simulink model "d_009_hvdc"  (Simulink 5.1)
settings: Solver=ode45  StartTime=0.0  StopTime=10.0  RelTol=1e-3
libraries: fm_lib x11
settings Model: Creator=fmilano  LastModifiedBy=fmilano  ExtModeAutoUpdateStatusClock=off  SignalLoggingName=logsout  RTWOptions="-aEnforceIntegerDowncast=1 -aFoldNonRolledExpr=1 -aInlineInvariantSignals=1 -aInlineParameters=0 -aLocalBlockOutputs=1 -aRollThreshold=5 -aZeroInternalMemoryAtStartup=1 -aZeroExternalMemoryAtStartup=1 -aInitFltsAndDblsToZero=1 -aForceBlockIOInitOptimize=0 -aGenerateReport=0 -aGenCodeOnly=0 -aRTWVerbose=1 -aIncludeHyperlinkInReport=0 -aLaunchReport=0 -aGenerateTraceInfo=0  -aForceParamTrailComments=0 -aGenerateComments=1 -aIgnoreCustomStorageClasses=1 -aIncHierarchyInIds=0 -aMaxRTWIdLen=31 -aShowEliminatedStatements=0 -aIncDataTypeInIds=0 -aInsertBlockDesc=0 -aIgnoreTestpoints=0 -aSimulinkBlockComments=1 -aInlinedPrmAccess=\"Literals\"  -aSuppressErrorStatus=0 -aModelReferenceCompliant=1 -aParenthesesLevel=\"Nominal\" -aModelStepFunctionPrototypeControlCompliant=0 -aPortableWordSizes=0 -aParMdlRefBuildCompliant=1 -aSupportNonInlinedSFcns=1 -aSupportContinuousTime=1 -aSupportComplex=1 -aSupportNonFinite=1 -aSupportAbsoluteTime=1 -aMultiwordLength=2048 -aTargetPreCompLibLocation=\"\" -aTargetLibSuffix=\"\" -aTargetFunctionLibrary=\"ANSI_C\" -aTargetFcnLib=\"ansi_tfl_tmw.mat\" -aMultiInstanceERTCode=0 -aLogVarNameModifier=\"rt_\" -aERTFirstTimeCompliant=0 -aIsPILTarget=0 -aCombineOutputUpdateFcns=0 -aGenerateASAP2=0 -aGenerateClassInterface=0 -aGenerateTestInterfaces=0 -aGenerateSampleERTMain=0 -aGenerateFullHeader=1 -aUtilityFuncGeneration=\"Auto\" -aIncludeFileDelimiter=\"Auto\" -aIncludeMdlTerminateFcn=1 -aPurelyIntegerCode=0 -aAutosarCompliant=0 -aERTCustomFileBanners=0 -aRTWCAPIStates=0 -aRTWCAPIParams=0 -aRTWCAPISignals=0 -aMatFileLogging=1 -aCompOptLevelCompliant=0 -aCPPClassGenCompliant=0 -aExtModeIntrfLevel=\"Level1\" -aExtModeMexFile=\"ext_comm\" -aExtModeTransport=0 -aExtModeStaticAllocSize=1000000 -aExtModeTesting=0 -aExtModeStaticAlloc=0 -aExtMode=0 -aERTMultiwordLength=256 -aERTMultiwordTypeDef=\"System defined\"  -aGenerateTraceInfo=0 -aIgnoreTestpoints=0 -aGenerateTraceInfo=0 -aGenerateTraceInfo=0 -aGenerateTraceInfo=0 -aGenerateTraceInfo=0 -aPrefixModelToSubsysFcnNames=1"

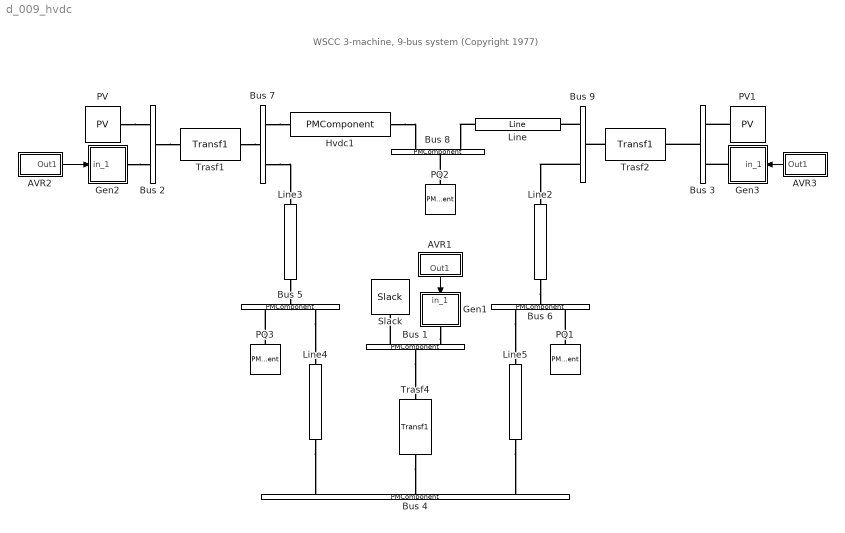
== system d_009_hvdc ==
  note: WSCC 3-machine, 9-bus system (Copyright 1977)
  AVR1 : Subsystem  Tag=PSATblock  Description=Controls  Orientation=down  mask(Exc){p2q=2, p3q=5.00, p4q=-5.00, p5q=20, p6q=0.2, p7q=0.063, p8q=0.35, p9q=1, p10q=0.314, p11q=0.001, p12_13q=[0.0039  1.555], in=0}
      mask prompts: p2q "Automatic Voltage Regulator Type"; p3q "Maximum Regulator Voltage [p.u.]"; p4q "Minimum Regulator Voltage [p.u.]"; p5q "Amplifier Gain Ka [p.u./p.u.]"; p6q "Amplifier Time Constant Ta [s]"; p7q "Stabilizer Gain Kf [p.u./p.u.]"; p8q "Stabilizer Time Tf [s]"; p9q "Integral deviation Ke [p.u./p.u.]"; p10q "Time Constant of the Field Circuit Td [s]"; p11q "Time Delay of the Measurement System Tr [s]"; p12_13q "Coefficient of the Ceiling Function (A B)"; in "Number of input signals"
      mask help: This block defines an Automatic Voltage Regulator.
      mask init:
      | fm_inout
      | [x,y] = fm_draw('R');
      mask Help:
      | This block defines an Automatic Voltage Regulator.
      | There are three kind of regulators:
      | 
      | Type 1:
      | 
      |      IEEE Model 1
      | 
      | Type 2:
      | 
      |      IEEE Model 2
      | 
      | Type 3:
      | 
      |      IEEE Model 3
      mask StyleString: popup(1|2|3),edit,edit,edit,edit,edit,edit,edit,edit,edit,edit,popup(0|1|2|3)
      mask CallbackString: fm_block|||||||||||
      mask Display:
      | plot([-1.8 4.1 4.1 -1.8 -1.8],[-1.5 -1.5 1.5 1.5 -1.5])
      | color('red')
      | plot([-1.3 -0.5],[-1 1],[-0.5 0.3],[1 -1],[-0.9 -0.1],[0.0 0.0])
      | plot(2.8+1.3*x,2*y,1.5+[-1.3 -0.5],[1 -1],1.5+[-0.5 0.3],[-1 1])
  AVR2 : Subsystem  Tag=PSATblock  Description=Controls  mask(Exc){p2q=2, p3q=5.00, p4q=-5.00, p5q=20, p6q=0.2, p7q=0.063, p8q=0.35, p9q=1, p10q=0.314, p11q=0.001, p12_13q=[0.0039  1.555], in=0}
      mask prompts: p2q "Automatic Voltage Regulator Type"; p3q "Maximum Regulator Voltage [p.u.]"; p4q "Minimum Regulator Voltage [p.u.]"; p5q "Amplifier Gain Ka [p.u./p.u.]"; p6q "Amplifier Time Constant Ta [s]"; p7q "Stabilizer Gain Kf [p.u./p.u.]"; p8q "Stabilizer Time Tf [s]"; p9q "Integral deviation Ke [p.u./p.u.]"; p10q "Time Constant of the Field Circuit Td [s]"; p11q "Time Delay of the Measurement System Tr [s]"; p12_13q "Coefficient of the Ceiling Function (A B)"; in "Number of input signals"
      mask help: This block defines an Automatic Voltage Regulator.
      mask init:
      | fm_inout
      | [x,y] = fm_draw('R');
      mask Help:
      | This block defines an Automatic Voltage Regulator.
      | There are three kind of regulators:
      | 
      | Type 1:
      | 
      |      IEEE Model 1
      | 
      | Type 2:
      | 
      |      IEEE Model 2
      | 
      | Type 3:
      | 
      |      IEEE Model 3
      mask StyleString: popup(1|2|3),edit,edit,edit,edit,edit,edit,edit,edit,edit,edit,popup(0|1|2|3)
      mask CallbackString: fm_block|||||||||||
      mask Display:
      | plot([-1.8 4.1 4.1 -1.8 -1.8],[-1.5 -1.5 1.5 1.5 -1.5])
      | color('red')
      | plot([-1.3 -0.5],[-1 1],[-0.5 0.3],[1 -1],[-0.9 -0.1],[0.0 0.0])
      | plot(2.8+1.3*x,2*y,1.5+[-1.3 -0.5],[1 -1],1.5+[-0.5 0.3],[-1 1])
  AVR3 : Subsystem  Tag=PSATblock  Description=Controls  Orientation=left  mask(Exc){p2q=2, p3q=5.00, p4q=-5.00, p5q=20, p6q=0.2, p7q=0.063, p8q=0.35, p9q=1, p10q=0.314, p11q=0.001, p12_13q=[0.0039  1.555], in=0}
      mask prompts: p2q "Automatic Voltage Regulator Type"; p3q "Maximum Regulator Voltage [p.u.]"; p4q "Minimum Regulator Voltage [p.u.]"; p5q "Amplifier Gain Ka [p.u./p.u.]"; p6q "Amplifier Time Constant Ta [s]"; p7q "Stabilizer Gain Kf [p.u./p.u.]"; p8q "Stabilizer Time Tf [s]"; p9q "Integral deviation Ke [p.u./p.u.]"; p10q "Time Constant of the Field Circuit Td [s]"; p11q "Time Delay of the Measurement System Tr [s]"; p12_13q "Coefficient of the Ceiling Function (A B)"; in "Number of input signals"
      mask help: This block defines an Automatic Voltage Regulator.
      mask init:
      | fm_inout
      | [x,y] = fm_draw('R');
      mask Help:
      | This block defines an Automatic Voltage Regulator.
      | There are three kind of regulators:
      | 
      | Type 1:
      | 
      |      IEEE Model 1
      | 
      | Type 2:
      | 
      |      IEEE Model 2
      | 
      | Type 3:
      | 
      |      IEEE Model 3
      mask StyleString: popup(1|2|3),edit,edit,edit,edit,edit,edit,edit,edit,edit,edit,popup(0|1|2|3)
      mask CallbackString: fm_block|||||||||||
      mask Display:
      | plot([-1.8 4.1 4.1 -1.8 -1.8],[-1.5 -1.5 1.5 1.5 -1.5])
      | color('red')
      | plot([-1.3 -0.5],[-1 1],[-0.5 0.3],[1 -1],[-0.9 -0.1],[0.0 0.0])
      | plot(2.8+1.3*x,2*y,1.5+[-1.3 -0.5],[1 -1],1.5+[-0.5 0.3],[-1 1])
  Bus 1 : PMComponent  Tag=PSATblock  Description=Connection  Orientation=down  PhysicalDomain=psatdomain  LeftPortType=p1  RightPortType=p1  LConnTagsString=__newl0|__newl1  RConnTagsString=__newr0  mask(Bus){in=2, out=1, p2q=16.5, p3_4q=[1.00   0.00], p5q=4, p6q=1}
      mask prompts: in "Number of inputs:"; out "Number of outputs:"; p2q "Voltage Rating [kV]"; p3_4q "Voltage initial guess [p.u.  rad]"; p5q "Area number"; p6q "Region number"
      mask help: Bus block.
      mask init:
      | fm_inout
      mask CallbackString: ||||fm_block|
      mask Display: plot([0 1 1 0 0],[0 0 1 1 0])
  Bus 2 : PMComponent  Tag=PSATblock  Description=Connection  PhysicalDomain=psatdomain  LeftPortType=p1  RightPortType=p1  LConnTagsString=__newl0|__newl1  RConnTagsString=__newr0  mask(Bus){in=2, out=1, p2q=18, p3_4q=[1.00   0.00], p5q=5, p6q=1}
      mask prompts: in "Number of inputs:"; out "Number of outputs:"; p2q "Voltage Rating [kV]"; p3_4q "Voltage initial guess [p.u.  rad]"; p5q "Area number"; p6q "Region number"
      mask help: Bus block.
      mask init:
      | fm_inout
      mask CallbackString: ||||fm_block|
      mask Display: plot([0 1 1 0 0],[0 0 1 1 0])
  Bus 3 : PMComponent  Tag=PSATblock  Description=Connection  Orientation=left  PhysicalDomain=psatdomain  LeftPortType=p1  RightPortType=p1  LConnTagsString=__newl0|__newl1  RConnTagsString=__newr0  mask(Bus){in=2, out=1, p2q=13.8, p3_4q=[1.00   0.00], p5q=3, p6q=1}
      mask prompts: in "Number of inputs:"; out "Number of outputs:"; p2q "Voltage Rating [kV]"; p3_4q "Voltage initial guess [p.u.  rad]"; p5q "Area number"; p6q "Region number"
      mask help: Bus block.
      mask init:
      | fm_inout
      mask CallbackString: ||||fm_block|
      mask Display: plot([0 1 1 0 0],[0 0 1 1 0])
  Bus 4 : PMComponent  Tag=PSATblock  Description=Connection  Orientation=down  PhysicalDomain=psatdomain  LeftPortType=p1  RightPortType=p1  LConnTagsString=__newl0|__newl1|__newl2  mask(Bus){in=3, out=0, p2q=230, p3_4q=[1.00   0.00], p5q=2, p6q=1}
      mask prompts: in "Number of inputs:"; out "Number of outputs:"; p2q "Voltage Rating [kV]"; p3_4q "Voltage initial guess [p.u.  rad]"; p5q "Area number"; p6q "Region number"
      mask help: Bus block.
      mask init:
      | fm_inout
      mask CallbackString: ||||fm_block|
      mask Display: plot([0 1 1 0 0],[0 0 1 1 0])
  Bus 5 : PMComponent  Tag=PSATblock  Description=Connection  Orientation=down  PhysicalDomain=psatdomain  LeftPortType=p1  RightPortType=p1  LConnTagsString=__newl0  RConnTagsString=__newr0|__newr1  mask(Bus){in=1, out=2, p2q=230, p3_4q=[1.00   0.00], p5q=2, p6q=1}
      mask prompts: in "Number of inputs:"; out "Number of outputs:"; p2q "Voltage Rating [kV]"; p3_4q "Voltage initial guess [p.u.  rad]"; p5q "Area number"; p6q "Region number"
      mask help: Bus block.
      mask init:
      | fm_inout
      mask CallbackString: ||||fm_block|
      mask Display: plot([0 1 1 0 0],[0 0 1 1 0])
  Bus 6 : PMComponent  Tag=PSATblock  Description=Connection  Orientation=down  PhysicalDomain=psatdomain  LeftPortType=p1  RightPortType=p1  LConnTagsString=__newl0  RConnTagsString=__newr0|__newr1  mask(Bus){in=1, out=2, p2q=230, p3_4q=[1.00   0.00], p5q=2, p6q=1}
      mask prompts: in "Number of inputs:"; out "Number of outputs:"; p2q "Voltage Rating [kV]"; p3_4q "Voltage initial guess [p.u.  rad]"; p5q "Area number"; p6q "Region number"
      mask help: Bus block.
      mask init:
      | fm_inout
      mask CallbackString: ||||fm_block|
      mask Display: plot([0 1 1 0 0],[0 0 1 1 0])
  Bus 7 : PMComponent  Tag=PSATblock  Description=Connection  PhysicalDomain=psatdomain  LeftPortType=p1  RightPortType=p1  LConnTagsString=__newl0  RConnTagsString=__newr0|__newr1  mask(Bus){in=1, out=2, p2q=230, p3_4q=[1.00   0.00], p5q=2, p6q=1}
      mask prompts: in "Number of inputs:"; out "Number of outputs:"; p2q "Voltage Rating [kV]"; p3_4q "Voltage initial guess [p.u.  rad]"; p5q "Area number"; p6q "Region number"
      mask help: Bus block.
      mask init:
      | fm_inout
      mask CallbackString: ||||fm_block|
      mask Display: plot([0 1 1 0 0],[0 0 1 1 0])
  Bus 8 : PMComponent  Tag=PSATblock  Description=Connection  Orientation=down  PhysicalDomain=psatdomain  LeftPortType=p1  RightPortType=p1  LConnTagsString=__newl0|__newl1  RConnTagsString=__newr0  mask(Bus){in=2, out=1, p2q=230, p3_4q=[1.00   0.00], p5q=2, p6q=1}
      mask prompts: in "Number of inputs:"; out "Number of outputs:"; p2q "Voltage Rating [kV]"; p3_4q "Voltage initial guess [p.u.  rad]"; p5q "Area number"; p6q "Region number"
      mask help: Bus block.
      mask init:
      | fm_inout
      mask CallbackString: ||||fm_block|
      mask Display: plot([0 1 1 0 0],[0 0 1 1 0])
  Bus 9 : PMComponent  Tag=PSATblock  Description=Connection  Orientation=left  PhysicalDomain=psatdomain  LeftPortType=p1  RightPortType=p1  LConnTagsString=__newl0  RConnTagsString=__newr0|__newr1  mask(Bus){in=1, out=2, p2q=230, p3_4q=[1.00   0.00], p5q=2, p6q=1}
      mask prompts: in "Number of inputs:"; out "Number of outputs:"; p2q "Voltage Rating [kV]"; p3_4q "Voltage initial guess [p.u.  rad]"; p5q "Area number"; p6q "Region number"
      mask help: Bus block.
      mask init:
      | fm_inout
      mask CallbackString: ||||fm_block|
      mask Display: plot([0 1 1 0 0],[0 0 1 1 0])
  Gen1 : Subsystem  Tag=PSATblock  Description=Machines  Orientation=down  mask(Syn){p2_3_4q=[100  16.5   60], p5q=4, p7_6q=[0.00  0.00], p8_9_10q=[0.1460  0.0608  0.0000], p11_12q=[8.96  0.00], p13_14_15q=[0.0969  0.0969  0.0000], p16_17q=[0.310  0.0000], p18_19q=[2*23.64  0.00], p20_21q=[0.00  0.00], p22_23q=[1.00  1.00], p24q=0.002, p25_26q=[0 0], in=1}
      mask prompts: p2_3_4q "Power, voltage and frequency ratings [MVA, kV, Hz]"; p5q "Machine Dynamic Order"; p7_6q "resistance ra and leakage reactance xl [p.u. p.u.]"; p8_9_10q "d-axis reactances Xd, X'd X"d [p.u.,p.u.,p.u.]"; p11_12q "d-axis open circuit time constants T'd0 and T"d0 [s, s]"; p13_14_15q "q-axis reactances Xq, X'q, X"q [p.u.  p.u.  p.u.]"; p16_17q "q-axis open circuit time constants T'q0 and T"q0 [s s]"; p18_19q "Inertia (M = 2H) and Damping [s, p.u.]"; p20_21q "Speed and active power additional signals Kw & Kp [p.u., p.u.]"; p22_23q "Percentage of active and reactive powers at bus [p.u. p.u.]"; p24q "d-axis additional circuit leakage time constant Taa [s]"; p25_26q "Saturation coefficients S(1.0) and S(1.2)"; in "Number of input signals"
      mask help: This block defines a fourth order synchronous machine.
      mask init:
      | fm_inout
      | [x,y] = fm_draw('circle');
      | [xg,yg] = fm_draw('G');
      | [xs,ys] = fm_draw('sinus');
      mask StyleString: edit,popup(8|6|5.3|5.2|5.1|4|3|2),edit,edit,edit,edit,edit,edit,edit,edit,edit,edit,popup(0|1|2)
      mask CallbackString: |fm_block|||||||||||
      mask Display:
      | plot(x+1.4,y,0.12*xs+1,0.15*ys-0.6)
      | color('blue')
      | plot(1.4+0.45*xg,0.3+0.45*yg)
  Gen2 : Subsystem  Tag=PSATblock  Description=Machines  mask(Syn){p2_3_4q=[100  18   60], p5q=4, p7_6q=[0.00  0.00], p8_9_10q=[0.8958  0.1198  0.0000], p11_12q=[6.00  0.00], p13_14_15q=[0.8645  0.1969  0.0000], p16_17q=[0.5350  0.0000], p18_19q=[12.80  0.00], p20_21q=[0.00  0.00], p22_23q=[1.00  1.00], p24q=0.002, p25_26q=[0 0], in=1}
      mask prompts: p2_3_4q "Power, voltage and frequency ratings [MVA, kV, Hz]"; p5q "Machine Dynamic Order"; p7_6q "resistance ra and leakage reactance xl [p.u. p.u.]"; p8_9_10q "d-axis reactances Xd, X'd X"d [p.u.,p.u.,p.u.]"; p11_12q "d-axis open circuit time constants T'd0 and T"d0 [s, s]"; p13_14_15q "q-axis reactances Xq, X'q, X"q [p.u.  p.u.  p.u.]"; p16_17q "q-axis open circuit time constants T'q0 and T"q0 [s s]"; p18_19q "Inertia (M = 2H) and Damping [s, p.u.]"; p20_21q "Speed and active power additional signals Kw & Kp [p.u., p.u.]"; p22_23q "Percentage of active and reactive powers at bus [p.u. p.u.]"; p24q "d-axis additional circuit leakage time constant Taa [s]"; p25_26q "Saturation coefficients S(1.0) and S(1.2)"; in "Number of input signals"
      mask help: This block defines a fourth order synchronous machine.
      mask init:
      | fm_inout
      | [x,y] = fm_draw('circle');
      | [xg,yg] = fm_draw('G');
      | [xs,ys] = fm_draw('sinus');
      mask StyleString: edit,popup(8|6|5.3|5.2|5.1|4|3|2),edit,edit,edit,edit,edit,edit,edit,edit,edit,edit,popup(0|1|2)
      mask CallbackString: |fm_block|||||||||||
      mask Display:
      | plot(x+1.4,y,0.12*xs+1,0.15*ys-0.6)
      | color('blue')
      | plot(1.4+0.45*xg,0.3+0.45*yg)
  Gen3 : Subsystem  Tag=PSATblock  Description=Machines  Orientation=left  mask(Syn){p2_3_4q=[100  13.8   60], p5q=4, p7_6q=[0.00  0.00], p8_9_10q=[1.3125  0.1813  0.0000], p11_12q=[5.89  0.00], p13_14_15q=[1.2578  0.2500  0.0000], p16_17q=[0.600  0.0000], p18_19q=[6.02  0.00], p20_21q=[0.00  0.00], p22_23q=[1.00  1.00], p24q=0.002, p25_26q=[0 0], in=1}
      mask prompts: p2_3_4q "Power, voltage and frequency ratings [MVA, kV, Hz]"; p5q "Machine Dynamic Order"; p7_6q "resistance ra and leakage reactance xl [p.u. p.u.]"; p8_9_10q "d-axis reactances Xd, X'd X"d [p.u.,p.u.,p.u.]"; p11_12q "d-axis open circuit time constants T'd0 and T"d0 [s, s]"; p13_14_15q "q-axis reactances Xq, X'q, X"q [p.u.  p.u.  p.u.]"; p16_17q "q-axis open circuit time constants T'q0 and T"q0 [s s]"; p18_19q "Inertia (M = 2H) and Damping [s, p.u.]"; p20_21q "Speed and active power additional signals Kw & Kp [p.u., p.u.]"; p22_23q "Percentage of active and reactive powers at bus [p.u. p.u.]"; p24q "d-axis additional circuit leakage time constant Taa [s]"; p25_26q "Saturation coefficients S(1.0) and S(1.2)"; in "Number of input signals"
      mask help: This block defines a fourth order synchronous machine.
      mask init:
      | fm_inout
      | [x,y] = fm_draw('circle');
      | [xg,yg] = fm_draw('G');
      | [xs,ys] = fm_draw('sinus');
      mask StyleString: edit,popup(8|6|5.3|5.2|5.1|4|3|2),edit,edit,edit,edit,edit,edit,edit,edit,edit,edit,popup(0|1|2)
      mask CallbackString: |fm_block|||||||||||
      mask Display:
      | plot(x+1.4,y,0.12*xs+1,0.15*ys-0.6)
      | color('blue')
      | plot(1.4+0.45*xg,0.3+0.45*yg)
  Hvdc1 : PMComponent  Tag=PSATblock  Description=FACTS  PhysicalDomain=psatdomain  LeftPortType=p1  RightPortType=p1  LConnTagsString=__newl0  RConnTagsString=__newr0  mask(Hvdc){p3_6q=[100  60], p4_5q=[230 230], p7_8q=[300 0.3], p9_10q=[0.1345   0.1257], p11_12q=[0.975  0.975], p13_14q=[20  25], p15_16q=[0.0625  0.200], p17_18q=[120  5], p19_20q=[40  18], p21_22_23_24q=[1.2   0.1  1.1  0.0], p25q=Current_control, p26_27_28q=[1  0.5  1.0], p29q=on}
      mask prompts: p3_6q "Power and Frequency Ratings [MVA,  Hz]"; p4_5q "Voltage Rating at Terminal Buses [kV, kV]"; p7_8q "DC Ratings (Vn_dc, In_dc) [kV, kA]"; p9_10q "Transformer Reactances (Xcr  Xci) [p.u.  p.u.]"; p11_12q "Tap Ratios (Ar Ai) [p.u./p.u.  p.u./p.u.]"; p13_14q "PI Regulator Constants (Ki, Kp)"; p15_16q "DC Line Parameters (Rdc Ldc) [p.u.  p.u.]"; p17_18q "Rectifier Angle Limits (a_max, a_min) [deg  deg]"; p19_20q "Inverter Angle Limits (g_max, g_min) [deg  deg]"; p21_22_23_24q "Reference dc voltage limits (Vr_max, Vr_min, Vi_max, Vi_min) [p.u.]"; p25q "Control type"; p26_27_28q "Current, active power and dc voltage orders [p.u.  p.u.  p.u.]"; p29q "Connected"
      mask help: This block defines a HVDC connection.
      mask init:
      | [x,y] = fm_draw('circle');
      mask StyleString: edit,edit,edit,edit,edit,edit,edit,edit,edit,edit,popup(Current_control|Power_control|Voltage_control),edit,checkbox
      mask CallbackString: ||||||||||||fm_block
      mask Display:
      | plot(0.7+[0 4 4 0 0],[-2 -2 2 2 -2])
      | plot(9.7+[0 4 4 0 0],[-2 -2 2 2 -2])
      | plot([4.7 9.7],[-1.25 -1.25],[4.7 9.7],[1.25 1.25])
      | 
      | plot(x-2,y,x-0.6,y,x+15,y,x+16.4,y)
      | color('green')
      | plot(-2+[-1 -1.3],[0 0],-2+[2.4 2.7],[0 0])
      | plot(-2+[-0.8 0.7],[-1.2 1.2],-2+[0.5 0.7],[1.1 1.2],-2+[0.7 0.7],[1.0 1.2])
      | plot(15+[-1 -1.3],[0 0],15+[2.4 2.7],[0 0])
      | plot(16.4+[-0.8 0.7],[-1.2 1.2],16.4+[0.5 0.7],[1.1 1.2],16.4+[0.7 0.7],[1.0 1.2])
      | 
      | color('magenta')
      | text(1.1,1.2,'R')
      | text(10.1,1.2,'I')
      | plot(0.7+[1 3 2 1],[-0.9 -0.9 0.9 -0.9])
      | plot(9.7+[1 3 2 1],[-0.9 -0.9 0.9 -0.9])
      | plot(0.7+[2 2],[0.9 1.25],0.7+[2 2],[-0.9 -1.25],0.7+[1.2 2.8],[0.9 0.9])
      | plot(9.7+[2 2],[0.9 1.25],9.7+[2 2],[-0.9 -1.25],9.7+[1.2 2.8],[0.9 0.9])
      | plot(0.7+[2 2.5],[0.9 1.25],9.7+[2 2.5],[0.9 1.25])
  Line : fm_lib/Power Flow/Line  Tag=PSATblock  Description=Power Flow  Orientation=left  PhysicalDomain=psatdomain  SubClassName=unknown  LeftPortType=p1  RightPortType=p1  LConnTagsString=__newl0  RConnTagsString=__newr0  p3_4_5q="[100  230  60]"  p6q=0  p8q=0.0119  p9q=0.1008  p10q=0.1045*2  p13_14_15q="[0.0  0.0  0.0]"  p16q=on
  Line2 : fm_lib/Power Flow/Line  Tag=PSATblock  Description=Power Flow  Orientation=down  PhysicalDomain=psatdomain  SubClassName=unknown  LeftPortType=p1  RightPortType=p1  LConnTagsString=__newl0  RConnTagsString=__newr0  p3_4_5q="[100  230  60]"  p6q=0  p8q=0.039  p9q=0.170  p10q=0.179*2  p13_14_15q="[0.0  0.0  0.0]"  p16q=on
  Line3 : fm_lib/Power Flow/Line  Tag=PSATblock  Description=Power Flow  Orientation=down  PhysicalDomain=psatdomain  SubClassName=unknown  LeftPortType=p1  RightPortType=p1  LConnTagsString=__newl0  RConnTagsString=__newr0  p3_4_5q="[100  230  60]"  p6q=0  p8q=0.032  p9q=0.161  p10q=0.153*2  p13_14_15q="[0.0  0.0  0.0]"  p16q=on
  Line4 : fm_lib/Power Flow/Line  Tag=PSATblock  Description=Power Flow  Orientation=down  PhysicalDomain=psatdomain  SubClassName=unknown  LeftPortType=p1  RightPortType=p1  LConnTagsString=__newl0  RConnTagsString=__newr0  p3_4_5q="[100  230  60]"  p6q=0  p8q=0.01  p9q=0.085  p10q=0.088*2  p13_14_15q="[0.0  0.0  0.0]"  p16q=on
  Line5 : fm_lib/Power Flow/Line  Tag=PSATblock  Description=Power Flow  Orientation=down  PhysicalDomain=psatdomain  SubClassName=unknown  LeftPortType=p1  RightPortType=p1  LConnTagsString=__newl0  RConnTagsString=__newr0  p3_4_5q="[100  230  60]"  p6q=0  p8q=0.017  p9q=0.092  p10q=0.079*2  p13_14_15q="[0.0  0.0  0.0]"  p16q=on
  PQ1 : PMComponent  Tag=PSATblock  Description=Power Flow  Orientation=down  PhysicalDomain=psatdomain  LeftPortType=p1  RightPortType=p1  LConnTagsString=__newl0  mask(PQ){p2_3q=[100  230], p4_5q=[0.90  0.30], p6_7q=[1.2  0.8], p8q=off, p9q=on}
      mask prompts: p2_3q "Power and Voltage Ratings [MVA, kV]"; p4_5q "Active and Reactive Powers [p.u.  p.u.]"; p6_7q "Maximum and Minimum Allowable Voltage [p.u.   p.u.]"; p8q "Allow conversion to impendance for min & max voltage"; p9q "Connected"
      mask help:
      | This block defines a constant power load:
      |
      | P = Pcost.
      | Q = Qcost.
      mask CallbackString: |||fm_block|fm_block
      mask Display: plot([1 -0.5 -0.5 1],[0 0.866 -0.866 0])
  PQ2 : PMComponent  Tag=PSATblock  Description=Power Flow  Orientation=down  PhysicalDomain=psatdomain  LeftPortType=p1  RightPortType=p1  LConnTagsString=__newl0  mask(PQ){p2_3q=[100  230], p4_5q=[1.00  0.35], p6_7q=[1.2  0.8], p8q=off, p9q=on}
      mask prompts: p2_3q "Power and Voltage Ratings [MVA, kV]"; p4_5q "Active and Reactive Powers [p.u.  p.u.]"; p6_7q "Maximum and Minimum Allowable Voltage [p.u.   p.u.]"; p8q "Allow conversion to impendance for min & max voltage"; p9q "Connected"
      mask help:
      | This block defines a constant power load:
      |
      | P = Pcost.
      | Q = Qcost.
      mask CallbackString: |||fm_block|fm_block
      mask Display: plot([1 -0.5 -0.5 1],[0 0.866 -0.866 0])
  PQ3 : PMComponent  Tag=PSATblock  Description=Power Flow  Orientation=down  PhysicalDomain=psatdomain  LeftPortType=p1  RightPortType=p1  LConnTagsString=__newl0  mask(PQ){p2_3q=[100  230], p4_5q=[1.25  0.50], p6_7q=[1.2  0.8], p8q=off, p9q=on}
      mask prompts: p2_3q "Power and Voltage Ratings [MVA, kV]"; p4_5q "Active and Reactive Powers [p.u.  p.u.]"; p6_7q "Maximum and Minimum Allowable Voltage [p.u.   p.u.]"; p8q "Allow conversion to impendance for min & max voltage"; p9q "Connected"
      mask help:
      | This block defines a constant power load:
      |
      | P = Pcost.
      | Q = Qcost.
      mask CallbackString: |||fm_block|fm_block
      mask Display: plot([1 -0.5 -0.5 1],[0 0.866 -0.866 0])
  PV : fm_lib/Power Flow/PV  Tag=PSATblock  Description=Power Flow  PhysicalDomain=psatdomain  SubClassName=unknown  LeftPortType=p1  RightPortType=p1  RConnTagsString=__newr0  p2_3q="[100  18]"  p4q=1.63  p5q=1.025  p6_7q=[99 -99]  p8_9q="[1.1  0.9]"  p10q=1  p11q=on
  PV1 : fm_lib/Power Flow/PV  Tag=PSATblock  Description=Power Flow  Orientation=left  PhysicalDomain=psatdomain  SubClassName=unknown  LeftPortType=p1  RightPortType=p1  RConnTagsString=__newr0  p2_3q="[100  13.8]"  p4q=0.85  p5q=1.025  p6_7q="[99  -99]"  p8_9q="[1.1  0.9]"  p10q=1  p11q=on
  Slack : fm_lib/Power Flow/Slack  Tag=PSATblock  Description=Power Flow  Orientation=down  PhysicalDomain=psatdomain  SubClassName=unknown  LeftPortType=p1  RightPortType=p1  RConnTagsString=__newr0  p2_3q="[100  16.5]"  p4q=1.04  p5q=0.00  p6_7q=[99 -99]  p8_9q="[1.1  0.9]"  p10q=0.80  p11q=1  p12q=on  p13q=on
  Trasf1 : fm_lib/Power Flow/Transf1  Tag=PSATblock  Description=Power Flow  PhysicalDomain=psatdomain  SubClassName=unknown  LeftPortType=p1  RightPortType=p1  LConnTagsString=__newl0  RConnTagsString=__newr0  p3_4_5q="[100  18  60]"  p7q=18/230  p8q=0.0  p9q=0.0625  p13_14_15q="[0.0  0.0  0.0]"  p16q=on
  Trasf2 : fm_lib/Power Flow/Transf1  Tag=PSATblock  Description=Power Flow  Orientation=left  PhysicalDomain=psatdomain  SubClassName=unknown  LeftPortType=p1  RightPortType=p1  LConnTagsString=__newl0  RConnTagsString=__newr0  p3_4_5q="[100  13.8  60]"  p7q=13.8/230  p8q=0.0  p9q=0.0586  p13_14_15q="[0.0  0.0  0.0]"  p16q=on
  Trasf4 : fm_lib/Power Flow/Transf1  Tag=PSATblock  Description=Power Flow  Orientation=down  PhysicalDomain=psatdomain  SubClassName=unknown  LeftPortType=p1  RightPortType=p1  LConnTagsString=__newl0  RConnTagsString=__newr0  p3_4_5q="[100  16.5  60]"  p7q=16.5/230  p8q=0.0  p9q=0.0576  p13_14_15q="[0.0  0.0  0.0]"  p16q=on
  wires:
  AVR2/1(Out1) -> Gen2/1(in_1)
  AVR3/1(Out1) -> Gen3/1(in_1)
  AVR1/1(Out1) -> Gen1/1(in_1)
  connections:
  Bus 7/RConn2 -- Line3/LConn1
  Gen1/RConn1 -- Bus 1/LConn2
  Gen3/RConn1 -- Bus 3/LConn2
  Gen2/RConn1 -- Bus 2/LConn2
  Bus 1/RConn1 -- Trasf4/LConn1
  Trasf4/RConn1 -- Bus 4/LConn2
  Line5/RConn1 -- Bus 4/LConn3
  Line4/RConn1 -- Bus 4/LConn1
  Bus 5/RConn2 -- Line4/LConn1
  Bus 6/RConn1 -- Line5/LConn1
  Line3/RConn1 -- Bus 5/LConn1
  Line2/RConn1 -- Bus 6/LConn1
  Bus 9/RConn2 -- Line2/LConn1
  Line/RConn1 -- Bus 8/LConn2
  Bus 7/RConn1 -- Hvdc1/LConn1
  Bus 9/RConn1 -- Line/LConn1
  Trasf2/RConn1 -- Bus 9/LConn1
  Trasf1/RConn1 -- Bus 7/LConn1
  Bus 3/RConn1 -- Trasf2/LConn1
  Bus 2/RConn1 -- Trasf1/LConn1
  PV1/RConn1 -- Bus 3/LConn1
  PV/RConn1 -- Bus 2/LConn1
  PQ1/LConn1 -- Bus 6/RConn2
  PQ2/LConn1 -- Bus 8/RConn1
  PQ3/LConn1 -- Bus 5/RConn1
  Bus 1/LConn1 -- Slack/RConn1
  Hvdc1/RConn1 -- Bus 8/LConn1

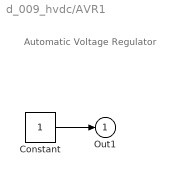
== system d_009_hvdc/AVR1 ==
  note: Automatic Voltage Regulator
  Constant : Constant  OutDataType=sfix(16)  OutScaling=2^0
  Out1 : Outport
  wires:
  Constant/1 -> Out1/1

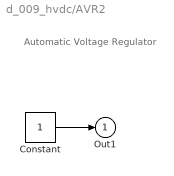
== system d_009_hvdc/AVR2 ==
  note: Automatic Voltage Regulator
  Constant : Constant  OutDataType=sfix(16)  OutScaling=2^0
  Out1 : Outport
  wires:
  Constant/1 -> Out1/1

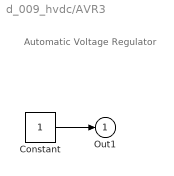
== system d_009_hvdc/AVR3 ==
  note: Automatic Voltage Regulator
  Constant : Constant  OutDataType=sfix(16)  OutScaling=2^0
  Out1 : Outport
  wires:
  Constant/1 -> Out1/1

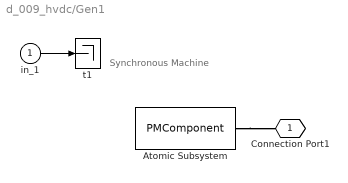
== system d_009_hvdc/Gen1 ==
  note: Synchronous Machine
  in_1 : Inport  OutDataType=sfix(16)  OutScaling=2^0
  Atomic Subsystem : PMComponent  PhysicalDomain=psatdomain  LeftPortType=p1  RightPortType=p1  RConnTagsString=__newr0
  t1 : Terminator
  Connection Port1 : PMIOPort  Tag=PMCPort  Orientation=left  Port=1  Side=Right
  wires:
  in_1/1 -> t1/1
  connections:
  Atomic Subsystem/RConn1 -- Connection Port1/RConn1

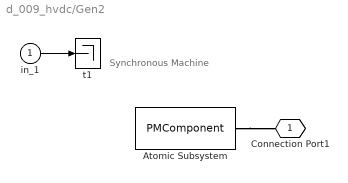
== system d_009_hvdc/Gen2 ==
  note: Synchronous Machine
  in_1 : Inport  OutDataType=sfix(16)  OutScaling=2^0
  Atomic Subsystem : PMComponent  PhysicalDomain=psatdomain  LeftPortType=p1  RightPortType=p1  RConnTagsString=__newr0
  t1 : Terminator
  Connection Port1 : PMIOPort  Tag=PMCPort  Orientation=left  Port=1  Side=Right
  wires:
  in_1/1 -> t1/1
  connections:
  Atomic Subsystem/RConn1 -- Connection Port1/RConn1

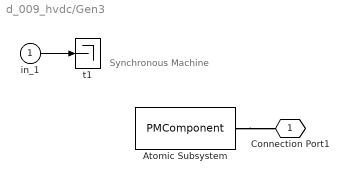
== system d_009_hvdc/Gen3 ==
  note: Synchronous Machine
  in_1 : Inport  OutDataType=sfix(16)  OutScaling=2^0
  Atomic Subsystem : PMComponent  PhysicalDomain=psatdomain  LeftPortType=p1  RightPortType=p1  RConnTagsString=__newr0
  t1 : Terminator
  Connection Port1 : PMIOPort  Tag=PMCPort  Orientation=left  Port=1  Side=Right
  wires:
  in_1/1 -> t1/1
  connections:
  Atomic Subsystem/RConn1 -- Connection Port1/RConn1
